simulink model "mimo1"  (Simulink 3.00)
settings: Solver=ode45  SolverMode=SingleTasking  StartTime=0.0  StopTime=20  MaxStep=0.010  RelTol=1e-3  AbsTol=1e-3
settings Model: TimeSaveName=t  SaveOutput=off

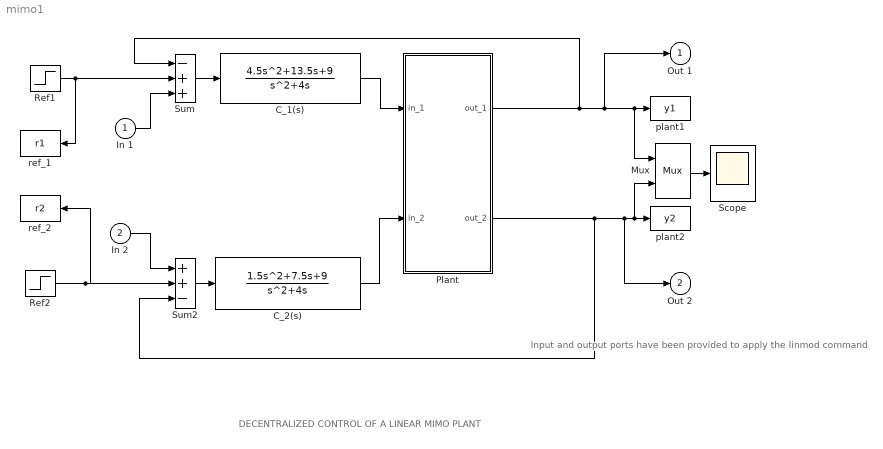
== system mimo1 ==
  note: DECENTRALIZED CONTROL OF A LINEAR MIMO PLANT
  note: Input and output ports
      | have been provided to apply
      | the linmod command
  In 1 : Inport  Port=1  PortWidth=-1  SampleTime=-1  DataType=auto
      settings: SignalType=auto
  In 2 : Inport  Port=2  PortWidth=-1  SampleTime=-1  DataType=auto
      settings: SignalType=auto
  C_1(s) : TransferFcn  Numerator=[4.5 13.5 9]  Denominator=[1 4 0]
  C_2(s) : TransferFcn  Numerator=[1.5 7.5 9]  Denominator=[1 4 0]
  Mux : Mux  Inputs=2
      settings: DisplayOption=none
  Plant : Subsystem
      mask Type: PLANT
      mask Display: disp('Plant')
  Ref1 : Step  Time=1  Before=0  After=1  SampleTime=0
  Ref2 : Step  Time=10  Before=0  After=-1  SampleTime=0
  Scope : Scope
      settings: TickLabels=on  TimeRange=20.000000  YMin=-4  YMax=4  SaveToWorkspace=off  SaveName=ScopeData  DataFormat=Matrix
  Sum : Sum  Inputs=-++  SaturateOnIntegerOverflow=on
  Sum2 : Sum  Inputs=++-  SaturateOnIntegerOverflow=on
  plant1 : ToWorkspace  VariableName=y1  SampleTime=0  SaveFormat=Matrix
      settings: Buffer=10000
  plant2 : ToWorkspace  VariableName=y2  SampleTime=0  SaveFormat=Matrix
      settings: Buffer=10000
  ref_1 : ToWorkspace  VariableName=r1  SampleTime=0  SaveFormat=Matrix
      settings: Buffer=10000
  ref_2 : ToWorkspace  VariableName=r2  SampleTime=0  SaveFormat=Matrix
      settings: Buffer=10000
  Out 1 : Outport  Port=1  InitialOutput=0
  Out 2 : Outport  Port=2  InitialOutput=0
  wires:
  Sum/1 -> C_1(s)/1
  C_1(s)/1 -> Plant/1(in_1)
  Sum2/1 -> C_2(s)/1
  Mux/1 -> Scope/1
  Ref1/1 -> Sum/2, ref_1/1
  Ref2/1 -> ref_2/1, Sum2/2
  In 2/1 -> Sum2/1
  In 1/1 -> Sum/3
  C_2(s)/1 -> Plant/2(in_2)
  Plant/1(out_1) -> Out 1/1, plant1/1, Mux/1, Sum/1
  Plant/2(out_2) -> Out 2/1, plant2/1, Mux/2, Sum2/3

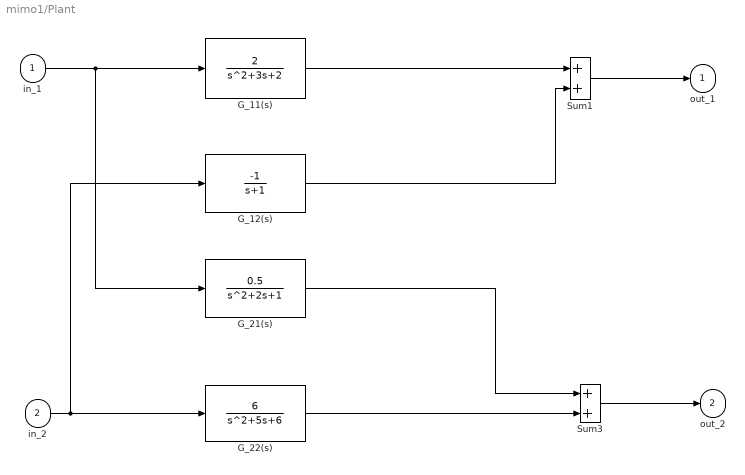
== system mimo1/Plant ==
  in_1 : Inport  Port=1  PortWidth=-1  SampleTime=-1  DataType=auto
      settings: SignalType=auto
  in_2 : Inport  Port=2  PortWidth=-1  SampleTime=-1  DataType=auto
      settings: SignalType=auto
  G_11(s) : TransferFcn  Numerator=2  Denominator=[1 3 2]
  G_12(s) : TransferFcn  Numerator=-1  Denominator=[1 1]
  G_21(s) : TransferFcn  Numerator=0.5  Denominator=[1 2 1]
  G_22(s) : TransferFcn  Numerator=[6]  Denominator=[1 5 6]
  Sum1 : Sum  Inputs=++  SaturateOnIntegerOverflow=on
  Sum3 : Sum  Inputs=++  SaturateOnIntegerOverflow=on
  out_1 : Outport  Port=1  InitialOutput=0
  out_2 : Outport  Port=2  InitialOutput=0
  wires:
  G_12(s)/1 -> Sum1/2
  G_11(s)/1 -> Sum1/1
  G_21(s)/1 -> Sum3/1
  G_22(s)/1 -> Sum3/2
  in_1/1 -> G_11(s)/1, G_21(s)/1
  in_2/1 -> G_22(s)/1, G_12(s)/1
  Sum1/1 -> out_1/1
  Sum3/1 -> out_2/1
